simulink model "gen_sim_model_speed"  (Simulink 10.1)
settings: Solver=ode45  StartTime=0  StopTime=10  FixedStep=0.01  RelTol=0.001  EnableMultiTasking=on
libraries: fmu_me_lib x1
settings Model: Creator=Tin Rabuzin  LastModifiedBy=meagh
settings DataIOCC: LimitDataPoints=on  OutputSaveName=simout  OutputOption=SpecifiedOutputTimes  OutputTimes=[0:0.01:10]
settings OptimizationCC: ExpressionDepthLimit=2147483647
settings DebuggingCC: SolverPrmCheckMsg=warning  StateNameClashWarn=warning
settings GRTTargetCC: CombineOutputUpdateFcns=on  GRTInterface=off

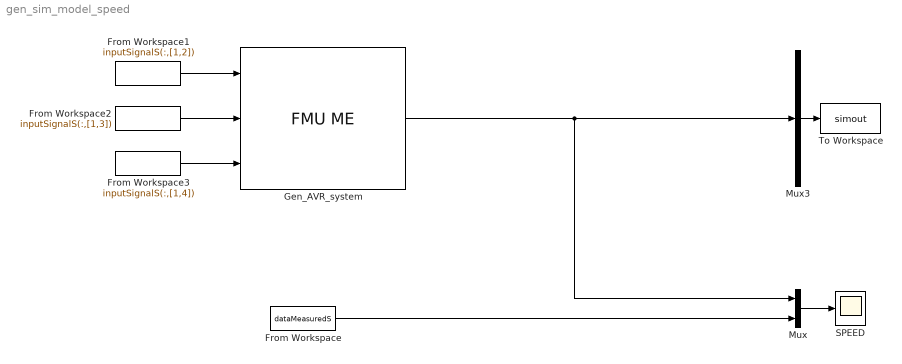
== system gen_sim_model_speed ==
  From Workspace : FromWorkspace  VariableName=dataMeasuredS
  From Workspace1 : FromWorkspace  VariableName=inputSignalS(:,[1,2])
  From Workspace2 : FromWorkspace  VariableName=inputSignalS(:,[1,3])
  From Workspace3 : FromWorkspace  VariableName=inputSignalS(:,[1,4])
  Gen_AVR_system : fmu_me_lib/FMU ME  Description=Simulates an FMU for Model Exchange 1.0 or Model Exchange 2.0.  dummy=0
  Mux : Mux  Inputs=2
  Mux3 : Mux  Inputs=1
  SPEED : Scope
  To Workspace : ToWorkspace  VariableName=simout  SaveFormat=Structure With Time  SampleTime=-1
  wires:
  Mux3/1 -> To Workspace/1
  Mux/1 -> SPEED/1
  From Workspace1/1 -> Gen_AVR_system/1
  From Workspace2/1 -> Gen_AVR_system/2
  From Workspace3/1 -> Gen_AVR_system/3
  Gen_AVR_system/1 -> Mux/1, Mux3/1
  From Workspace/1 -> Mux/2
